simulink model "prob11"  (R2013a)
settings: Solver=ode23s  StartTime=0.0  StopTime=10.0  RelTol=1e-3
libraries: fl_lib x13, nesl_utility x4, simulink x2
settings Model: Creator=Suddenlink  LastModifiedBy=Suddenlink

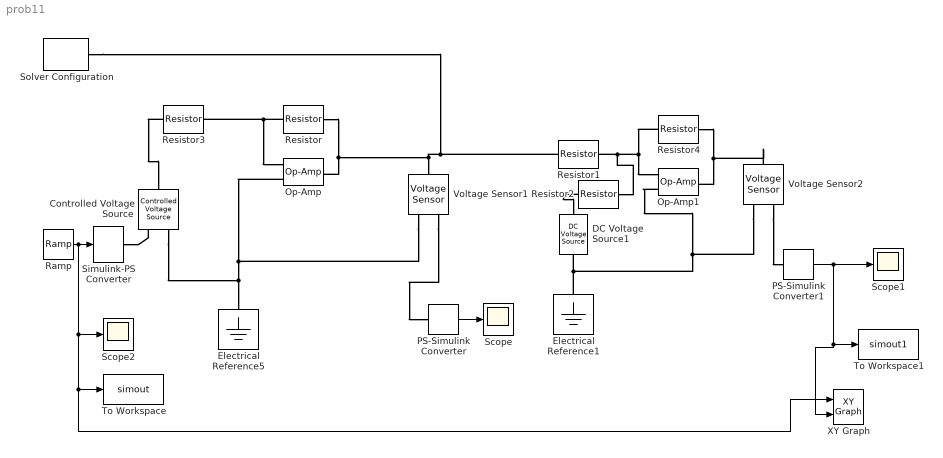
== system prob11 ==
  Controlled Voltage Source : fl_lib/Electrical/Electrical Sources/Controlled Voltage Source  i_Log=off  v_Log=off  LocalVarNames=|i|v  LocalVarDescs=|i|v  LocalVarLogging=[0 0]
  DC Voltage Source1 : fl_lib/Electrical/Electrical Sources/DC Voltage Source  v0=-0.32 V  i_Log=off  v_Log=off  LocalVarNames=|i|v  LocalVarDescs=|i|v  LocalVarLogging=[0 0]
  Electrical Reference1 : fl_lib/Electrical/Electrical Elements/Electrical Reference  i_Log=off  LocalVarNames=|i  LocalVarDescs=|i  LocalVarLogging=0
  Electrical Reference5 : fl_lib/Electrical/Electrical Elements/Electrical Reference  i_Log=off  LocalVarNames=|i  LocalVarDescs=|i  LocalVarLogging=0
  Op-Amp : fl_lib/Electrical/Electrical Elements/Op-Amp  i1_Log=off  v1_Log=off  outI_Log=off  LocalVarNames=|i1|v1|outI  LocalVarDescs=|i1|v1|outI  LocalVarLogging=[0 0 0]
  Op-Amp1 : fl_lib/Electrical/Electrical Elements/Op-Amp  i1_Log=off  v1_Log=off  outI_Log=off  LocalVarNames=|i1|v1|outI  LocalVarDescs=|i1|v1|outI  LocalVarLogging=[0 0 0]
  PS-Simulink Converter : nesl_utility/PS-Simulink Converter  PhysicalDomain=network_engine_domain  SubClassName=ps_output  LeftPortType=input  RightPortType=output  PseudoPeriodic=off  Frequencies=[]  Unit=1  AffineConversion=off
  PS-Simulink Converter1 : nesl_utility/PS-Simulink Converter  PhysicalDomain=network_engine_domain  SubClassName=ps_output  LeftPortType=input  RightPortType=output  PseudoPeriodic=off  Frequencies=[]  Unit=1  AffineConversion=off
  Ramp : simulink/Sources/Ramp  slope=0.1  start=0  X0=0
  Resistor : fl_lib/Electrical/Electrical Elements/Resistor  R=1800 Ohm  i_Log=off  v_Log=off  LocalVarNames=|i|v  LocalVarDescs=|i|v  LocalVarLogging=[0 0]
  Resistor{1..4} (4 alike) : fl_lib/Electrical/Electrical Elements/Resistor  R=1000 Ohm  i_Log=off  v_Log=off  LocalVarNames=|i|v  LocalVarDescs=|i|v  LocalVarLogging=[0 0]
  Scope : Scope
  Scope1 : Scope
  Scope2 : Scope
      settings: SaveName=ScopeData2
  Simulink-PS Converter : nesl_utility/Simulink-PS Converter  PhysicalDomain=network_engine_domain  SubClassName=ps_input  LeftPortType=input  RightPortType=output  PseudoPeriodic=off  Frequencies=[]  NoiseDistribution=none  NoiseParameters=[]  Unit=1  AffineConversion=off  InputFiltering=off  SimscapeFilterOrder=1  InputFilterTimeConstant=0.001  UdotUserProvided=1
  Solver Configuration : nesl_utility/Solver Configuration  PhysicalDomain=network_engine_domain  SubClassName=solver  LeftPortType=input  RightPortType=generic  Accelerate=off  Tones=[]  Harmonics=[]  SimulateNoise=off  Profile=off  UseLocalSampling=off  EnableSwitchedLinearOptims=on  FrequencyDomain=off  UseCCode=off  UseNewInitialization=off  DoDC=off  ResidualTolerance=1e-09  UseLocalSolver=on  LocalSolverChoice=NE_TRAPEZOIDAL_ADVANCER  LocalSolverSampleTime=0.001  DoFixedCost=on  MaxNonlinIter=3  MaxModeIter=2  LinearAlgebra=Full  DelaysMemoryBudget=1024
  To Workspace : ToWorkspace  VariableName=simout  SampleTime=-1  SaveFormat=Timeseries
  To Workspace1 : ToWorkspace  VariableName=simout1  SampleTime=-1  SaveFormat=Timeseries
  Voltage Sensor1 : fl_lib/Electrical/Electrical Sensors/Voltage Sensor  i1_Log=off  v1_Log=off  LocalVarNames=|i1|v1  LocalVarDescs=|i1|v1  LocalVarLogging=[0 0]
  Voltage Sensor2 : fl_lib/Electrical/Electrical Sensors/Voltage Sensor  i1_Log=off  v1_Log=off  LocalVarNames=|i1|v1  LocalVarDescs=|i1|v1  LocalVarLogging=[0 0]
  XY Graph : simulink/Sinks/XY Graph  xmin=0  xmax=1  ymin=0  ymax=2.5  st=-1
      settings: AttributesFormatString=%<degF Vo vs deg C Vin>
  wires:
  PS-Simulink Converter/1 -> Scope/1
  PS-Simulink Converter1/1 -> XY Graph/2, To Workspace1/1, Scope1/1
  Ramp/1 -> XY Graph/1, To Workspace/1, Scope2/1, Simulink-PS Converter/1
  connections:
  Op-Amp/RConn1 -- Resistor/RConn1 -- Solver Configuration/RConn1 -- Resistor1/LConn1 -- Voltage Sensor1/LConn1
  Resistor/LConn1 -- Op-Amp/LConn2 -- Resistor3/RConn1
  Resistor3/LConn1 -- Controlled Voltage Source/LConn1
  Voltage Sensor1/RConn2 -- Controlled Voltage Source/RConn2 -- Electrical Reference5/LConn1 -- Op-Amp/LConn1
  Voltage Sensor1/RConn1 -- PS-Simulink Converter/LConn1
  Resistor4/RConn1 -- Voltage Sensor2/LConn1 -- Op-Amp1/RConn1
  Resistor4/LConn1 -- Resistor2/RConn1 -- Resistor1/RConn1 -- Op-Amp1/LConn2
  Electrical Reference1/LConn1 -- Voltage Sensor2/RConn2 -- Op-Amp1/LConn1 -- DC Voltage Source1/RConn1
  Resistor2/LConn1 -- DC Voltage Source1/LConn1
  Voltage Sensor2/RConn1 -- PS-Simulink Converter1/LConn1
  Simulink-PS Converter/RConn1 -- Controlled Voltage Source/RConn1
